simulink model "SPSA"  (R2020b)
settings: Solver=VariableStepAuto  StartTime=0.0  StopTime=10.0  RelTol=1e-3
undefined symbols (not defined in the file): binornd
settings Model: Creator=Arman  LastModifiedBy=Arman
settings DebuggingCC: UnconnectedInputMsg=none  UnconnectedOutputMsg=none  UnconnectedLineMsg=none
settings ModelReferenceCC: EnableRefExpFcnMdlSchedulingChecks=off

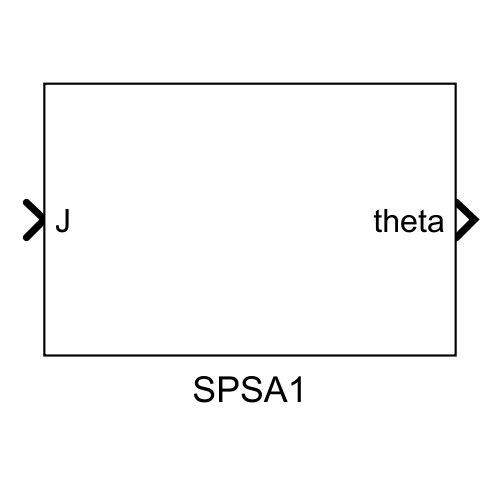
[thumbnail: Simulink's stored preview of the top-level diagram]
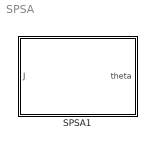
== system SPSA ==
  SPSA1 : Subsystem  SystemSampleTime=0.1  mask{c=0.01, gamma=0.101, alpha=0.1, AA=1, a=0.01, n=3, Ts=0.01, theta_0=[1,2,3], normThreshold=inf, eps=1e-6}
      mask prompts: AA "A"; n "n_vars"; Ts "Sample Time"; theta_0 "Initial Condition"; normThreshold "Gradient Norm Threshhold"; eps "epsilon"
      mask DialogControl ParameterGroupVar Prompt: solver parameter
      mask DialogControl Container3 Prompt: g1 parameter
      mask DialogControl Container4 Prompt: g2 Parameter

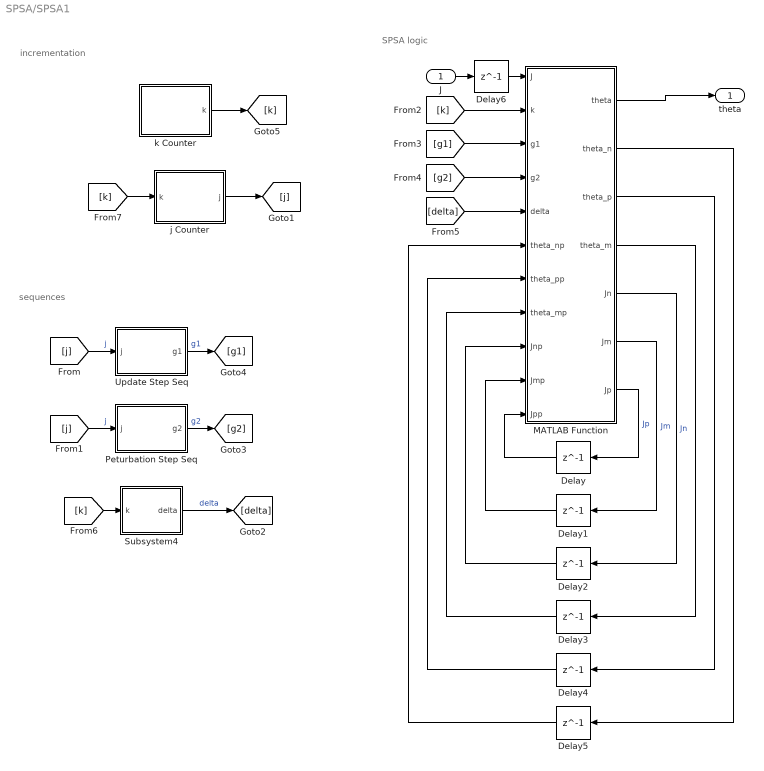
== system SPSA/SPSA1 ==
  note: SPSA logic
  note: incrementation
  note: sequences
  J : Inport
  Delay{,1..4} (5 alike) : Delay  DelayLength=1  SampleTime=Ts
  Delay5 : Delay  DelayLength=1  InitialCondition=theta_0  SampleTime=Ts
  Delay6 : Delay  DelayLength=1
  MATLAB Function : MATLAB Function  TreatAsAtomicUnit=on
  Peturbation Step Seq : Subsystem  mask{c=c, gamma=gamma}
  Subsystem4 : Subsystem  mask{n=n, Ts=Ts}
      mask prompts: n "n_vars"
  Update Step Seq : Subsystem  mask{a=a, AA=AA, alpha=alpha}
      mask prompts: AA "A"
  j Counter : Subsystem
  k Counter : Subsystem
  theta : Outport
  wires:
  J/1 -> Delay6/1
  MATLAB Function/1(theta) -> theta/1
  MATLAB Function/7(Jp) -> Delay/1  "Jp"
  Delay/1 -> MATLAB Function/11(Jpp)
  MATLAB Function/6(Jm) -> Delay1/1  "Jm"
  Delay1/1 -> MATLAB Function/10(Jmp)
  MATLAB Function/5(Jn) -> Delay2/1  "Jn"
  Delay2/1 -> MATLAB Function/9(Jnp)
  MATLAB Function/4(theta_m) -> Delay3/1
  Delay3/1 -> MATLAB Function/8(theta_mp)
  MATLAB Function/3(theta_p) -> Delay4/1
  Delay4/1 -> MATLAB Function/7(theta_pp)
  MATLAB Function/2(theta_n) -> Delay5/1
  Delay5/1 -> MATLAB Function/6(theta_np)
  [j] -> Update Step Seq/1(j)  "j"
  j Counter/1(j) -> [j]
  [j] -> Peturbation Step Seq/1(j)  "j"
  Subsystem4/1(delta) -> [delta]  "delta"
  Update Step Seq/1(g1) -> [g1]  "g1"
  Peturbation Step Seq/1(g2) -> [g2]  "g2"
  k Counter/1(k) -> [k]
  [k] -> MATLAB Function/2(k)
  [g1] -> MATLAB Function/3(g1)
  [g2] -> MATLAB Function/4(g2)
  [delta] -> MATLAB Function/5(delta)
  [k] -> Subsystem4/1(k)
  Delay6/1 -> MATLAB Function/1(J)
  [k] -> j Counter/1(k)

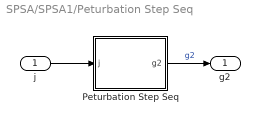
== system SPSA/SPSA1/Peturbation Step Seq ==
  j : Inport
  Peturbation Step Seq : MATLAB Function  TreatAsAtomicUnit=on
  g2 : Outport
  wires:
  Peturbation Step Seq/1(g2) -> g2/1  "g2"
  j/1 -> Peturbation Step Seq/1(j)

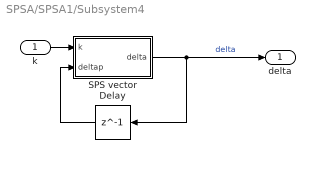
== system SPSA/SPSA1/Subsystem4 ==
  k : Inport
  Delay : Delay  DelayLength=1  InitialCondition=2*binornd(1,0.5,n,1)-1  SampleTime=Ts
  SPS vector : MATLAB Function  TreatAsAtomicUnit=on
  delta : Outport
  wires:
  SPS vector/1(delta) -> Delay/1, delta/1  "delta"
  Delay/1 -> SPS vector/2(deltap)
  k/1 -> SPS vector/1(k)

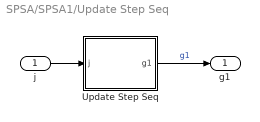
== system SPSA/SPSA1/Update Step Seq ==
  j : Inport
  Update Step Seq : MATLAB Function  TreatAsAtomicUnit=on
  g1 : Outport
  wires:
  j/1 -> Update Step Seq/1(j)
  Update Step Seq/1(g1) -> g1/1  "g1"

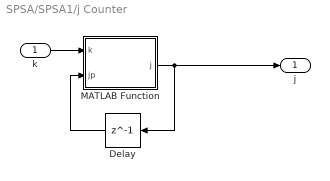
== system SPSA/SPSA1/j Counter ==
  k : Inport
  Delay : Delay  DelayLength=1
  MATLAB Function : MATLAB Function  TreatAsAtomicUnit=on
  j : Outport
  wires:
  MATLAB Function/1(j) -> j/1, Delay/1
  Delay/1 -> MATLAB Function/2(jp)
  k/1 -> MATLAB Function/1(k)

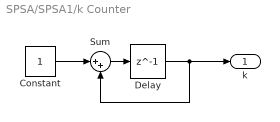
== system SPSA/SPSA1/k Counter ==
  Constant : Constant
  Delay : Delay  DelayLength=1  SampleTime=Ts
  Sum : Sum  Inputs=|++
  k : Outport
  wires:
  Sum/1 -> Delay/1
  Delay/1 -> k/1, Sum/2
  Constant/1 -> Sum/1

== matlab function SPSA/SPSA1/MATLAB Function ==
  data: J input; k input; g1 input; g2 input; delta input; theta_np input; theta_pp input; theta_mp input; Jnp input; Jmp input; Jpp input; theta output; theta_n output; theta_p output; theta_m output; n parameter; Jn output; Jm output; Jp output; normThreshold parameter; eps parameter
function [theta, theta_n,theta_p, theta_m,Jn, Jm, Jp] = fcn(J, k, g1, g2, delta, theta_np, theta_pp, theta_mp, Jnp, Jmp, Jpp, n, normThreshold, eps)
s = rem(k, 3);

theta = zeros(n,1);
theta_n = zeros(n,1);
theta_m = zeros(n,1);
theta_p = zeros(n,1);
Jn = 0;
Jp = 0;
Jm = 0;
switch s
    case 0
        % cost function assignment
        Jn = Jnp;
        Jm = J;
        Jp = Jpp;
        % gradient estimation
        sigma = (Jp-Jm)./(2*g2*delta+eps);
        
        % TODO: make gradient clipping optional
        nsig = norm(sigma);
        if nsig > normThreshold
            sigma = sigma*normThreshold/nsig;
        end

        % new theta
        theta_n= theta_np - g1*sigma;
        theta_m= theta_mp;
        theta_p= theta_pp;
        % output theta
        theta = theta_n;
    case 1
        % cost function assignment
        Jp = Jpp;
        Jn = J;
        Jm = Jmp;
        % new theta
        theta_n= theta_np;
        theta_m= theta_mp;
        theta_p= theta_np+g2*delta;

        % output theta
        theta = theta_p;
    case 2
        % cost function assignment
        Jm = Jmp;
        Jp = J;
        Jn = Jnp;
        % new theta
        theta_n= theta_np;
        theta_m= theta_np -g2*delta;
        theta_p= theta_pp;

        % output theta
        theta = theta_m;
    otherwise
end

== matlab function SPSA/SPSA1/Update Step Seq/Update Step Seq ==
  data: j input; g1 output; a parameter; AA parameter; alpha parameter
function g1 = fcn(j, a, AA, alpha)  
    g1 = a/(j+1+AA)^alpha;
end

== matlab function SPSA/SPSA1/Peturbation Step Seq/Peturbation Step Seq ==
  data: j input; g2 output; c parameter; gamma parameter
function g2 = fcn(j, c, gamma)
    g2 = c/(j+1)^gamma;
end

== matlab function SPSA/SPSA1/Subsystem4/SPS vector ==
  data: k input; deltap input; delta output; n parameter int32
function delta = fcn(k,deltap, n)
s = rem(k,3);
switch s
    case 1
        delta = binornd(1,0.5,n,1);
        delta = 2*delta-1;
    otherwise
        delta = deltap;
end

end

== matlab function SPSA/SPSA1/j Counter/MATLAB Function ==
  data: k input; j output; jp input
function j = fcn(k,jp)
s = rem(k,3);
switch s
    case 1
        j = jp+1;
    otherwise
        j = jp;
end
end
